simulink model "MultiAgentQUAV"  (R2017a)
settings: Solver=ode1  StartTime=0.0  StopTime=50  FixedStep=tstep  RelTol=1e-3
InitFcn:
  | initSim;
StopFcn:
  | plotSimSolution;
values from neighbouring files (symbols this model uses):
  N = cross(u,v)'    [MultiAgentQUAVPlantNewtOLD.m]    (also in MultiAgentQUAVProblemNewt.m = size(phi,1); initSim.m = 20)
  tstep = 0.1    [initSim.m]
undefined symbols (not defined in the file or in its folder): m, problem, X, Y, Z
libraries: nesl_utility x38, sm_lib x25, sharedtransform x4
(part 1 of 3)
settings Model: Creator=yn15  LastModifiedBy=daw15
settings OptimizationCC: LifeSpan=inf
settings DebuggingCC: SFUnexpectedBacktrackingDiag=warning  SFNoUnconditionalDefaultTransitionDiag=warning  SFExecutionAtInitializationDiag=none
settings GRTTargetCC: TargetLangStandard=C89/C90 (ANSI)
settings ConfigComp: CovMetricSettings=dw  CovHtmlReporting=on  CovSaveCumulativeToWorkspaceVar=on  CovSaveSingleToWorkspaceVar=on  CovExternalEMLEnable=off

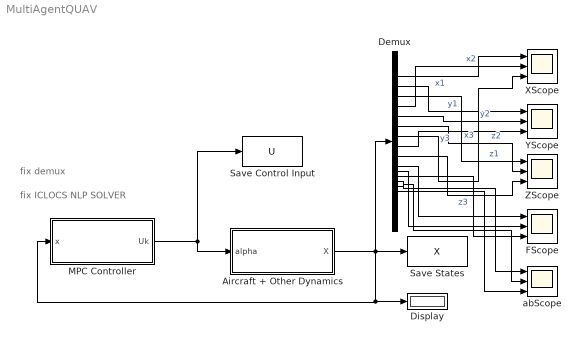
== system MultiAgentQUAV ==
  note: fix ICLOCS NLP SOLVER
  note: fix demux
  Aircraft + Other Dynamics : Subsystem
  Demux : Demux  Outputs=27
  Display : Display
  FScope : Scope  NumInputPorts=3
  "MPC Controller " : Subsystem
  Save Control Input : ToWorkspace  VariableName=U  SampleTime=-1
      settings: Save2DSignal=2-D array (concatenate along first dimension)
  Save States : ToWorkspace  VariableName=X  SaveFormat=Timeseries  SampleTime=-1
  XScope : Scope  NumInputPorts=3
  YScope : Scope  NumInputPorts=3
  ZScope : Scope  NumInputPorts=3
  abScope : Scope  NumInputPorts=3
  wires:
  Aircraft + Other Dynamics/1(X) -> Demux/1, Save States/1, "MPC Controller "/1(x), Display/1
  Demux/1 -> XScope/1  "x1"
  "MPC Controller "/1(Uk) -> Save Control Input/1, Aircraft + Other Dynamics/1(alpha)
  Demux/3 -> YScope/1  "y1"
  Demux/5 -> ZScope/1  "z1"
  Demux/7 -> XScope/2  "x2"
  Demux/9 -> YScope/2  "y2"
  Demux/11 -> ZScope/2  "z2"
  Demux/13 -> XScope/3  "x3"
  Demux/15 -> YScope/3  "y3"
  Demux/17 -> ZScope/3  "z3"
  Demux/19 -> FScope/1
  Demux/20 -> FScope/2
  Demux/21 -> FScope/3
  Demux/22 -> abScope/1
  Demux/23 -> abScope/2
  Demux/24 -> abScope/3
